simulink model "TVModel_Simulation_21"  (R2021b)
settings: Solver=FixedStepDiscrete  StartTime=0.0  StopTime=250  FixedStep=0.02  MaxStep=0.01  RelTol=1e-3
undefined symbols (not defined in the file or in its folder): MB, TV, TV_OLD
libraries: simulink x22, simulink_extras x14, eeGeneralControl x13, slpidlib x8, fuzblock x4, controlLib x4, cstblocks x3, dspstat3 x2, eeSlidingModeController x1, sharedTrackingLibrary x1
(part 7 of 9)

== matlab function TVModel_Simulation_21/Subsystem/Subsystem1/Torque Distribution/MPC/ PRE LUDO/Cross Check1 ==
  data: ubu input; param input; ubu output; lbu input; lbu output
function [ubu,lbu] = fcn(ubu,param,lbu)
flag = param(1);
ubu_target = param(2:5);
lbu_target = param(6:9);
lbu_max = param(10);
switch flag
    case 0 %% Check cross between bounds
        for i = 1 : 4
            if lbu(i) > ubu(i)
               lbu(i) = ubu(i) - lbu_max;
            end
        end
    case 1 %% Check for low YRD Accelerating
        for i = 1 :4
            ubu(i) = ubu_target(i);
            lbu(i) = 0;
        end
    case 2 %% Check for low YRD Braking
        for i = 1:4
            lbu(i) = lbu_target(i);
            ubu(i) = 0;
        end
    case 3 %% Overlapping
        for i = 1:4
            lbu(i) = 0;
            ubu(i) = 0;
        end
end

== matlab function TVModel_Simulation_21/Subsystem/Subsystem1/Torque Distribution/MPC/USEFUL STUFFFF/Extended Kalman Filter/state_update_kalman_simulink/f(x,u) ==
  data: x input; u input; xout output
function xout = state_update_kalman_simulink(x,u)

%% ~~~~~~~~~~~~~~~~~~~~~~~~~~~~~ Intro ~~~~~~~~~~~~~~~~~~~~~~~~~~~~~~~~~~~~
dt = 1/50;
%% ~~~~~~~~~~~~~~~~~~~~~~~~ Car parameters ~~~~~~~~~~~~~~~~~~~~~~~~~~~~~~~~
xout = zeros(3,1);
% ~~~~~~~~~~~~~~~~~~~~~~~~ General Parameters ~~~~~~~~~~~~~~~~~~~~~~~~~~~~~
g   = 9.81;            % [m/s^2]                          
wd  = 0.5;             % [~]         
wb  = 1.53;            % [~]          
tf  = 1.27;            % [m]          
tr  = 1.27;            % [m]          
m   = 195+75;          % [Kg]            
Iz  = 120;             % [Kg*m^2]         
a   = wb*wd;           % [m]            
b   = wb - a;          % [m]            
hcog = 0.29;           % [m]           
Fzf  = m*g/2*(wd);     % [N]                 
Fzr  = m*g/2*(1-wd);   % [N]                   
tau = 13.5;            % [~]          
rs  = 0.235;           % [m]           

% ~~~~~~~~~~~~~~~~~~~~~~~~~~~ Aero parameters ~~~~~~~~~~~~~~~~~~~~~~~~~~~~~
wbaero = 0.5542;       % [~]           
hcop = 0.576;          % [m]      
rho = 1.225;           % [Kg/m^3]     
CdA = 1.708;           % [m]     
ClA = 5.14;            % [m]    

% ~~~~~~~~~~~~~~~~~~~~~~~~~~ Other parameters ~~~~~~~~~~~~~~~~~~~~~~~~~~~~~

% ~~~~~~~~~~~~~~~~~~~~~~~~~~~ Set up states  ~~~~~~~~~~~~~~~~~~~~~~~~~~~~~~
vx = x(1);
vy = x(2);
r  = x(3);

% ~~~~~~~~~~~~~~~~~~~~~~~~~~~ Set up parameters ~~~~~~~~~~~~~~~~~~~~~~~~~~~
% delta    = u(1);
% kappa_FL = u(2);
% kappa_FR = u(3);
% kappa_RL = u(4);
% kappa_RR = u(5);
% Tbrk_FL  = u(6);
% Tbrk_FR  = u(7);
% Tbrk_RL  = u(8);
% Tbrk_RR  = u(9);
% ay       = u(10);
% ax       = u(11);
% T_FL     = u(12);
% T_FR     = u(13);
% T_RL     = u(14);
% T_RR     = u(15);

delta    = u(1);
kappa_FL = u(2);
kappa_FR = u(3);
kappa_RL = u(4);
kappa_RR = u(5);
T_FL     = u(6);
T_FR     = u(7);
T_RL     = u(8);
T_RR     = u(9);

ax = 0; ay = 0;
Tbrk_FL  = 0;
Tbrk_FR  = 0;
Tbrk_RL  = 0;
Tbrk_RR  = 0;
%% ~~~~~~~~~~~~~~~~~~~~~~~~~~ System Dynamics ~~~~~~~~~~~~~~~~~~~~~~~~~~~~~~

% ~~~~~~~~~~~~~~~~~~~~~~~~~~~ Aerodynamics ~~~~~~~~~~~~~~~~~~~~~~~~~~~~~~~~
Faerox = 0.5*rho*CdA*vx^2;
Faeroz = 0.5*rho*ClA*vx^2;

% ~~~~~~~~~~~~~~~~~~~~~~~~~~~ Slip Angles ~~~~~~~~~~~~~~~~~~~~~~~~~~~~~~~~~
alpha_FL =  (((vy + r*a)./(vx - r*tf/2)) - delta);
alpha_FR =  (((vy + r*a)./(vx + r*tf/2)) - delta);
alpha_RL =  (((vy - r*b)./(vx - r*tr/2)));     
alpha_RR =  (((vy - r*b)./(vx + r*tr/2)));     

% ~~~~~~~~~~~~~~~~~~~~~~~~~~~ Vertical loads ~~~~~~~~~~~~~~~~~~~~~~~~~~~~~~
Fz_FL = Fzf - 0.5*(m/tf*hcog).*ay + 0.5*Faeroz*wbaero - 0.5*Faerox/wb*hcop - 0.5*(m/wb*hcog).*ax;
Fz_FR = Fzf + 0.5*(m/tf*hcog).*ay + 0.5*Faeroz*wbaero - 0.5*Faerox/wb*hcop - 0.5*(m/wb*hcog).*ax;
Fz_RL = Fzr - 0.5*(m/tr*hcog).*ay + 0.5*Faeroz*(1-wbaero) + 0.5*Faerox/wb*hcop + 0.5*(m/wb*hcog).*ax;
Fz_RR = Fzr + 0.5*(m/tr*hcog).*ay + 0.5*Faeroz*(1-wbaero) + 0.5*Faerox/wb*hcop + 0.5*(m/wb*hcog).*ax;

% ~~~~~~~~~~~~~~~~~~~~~~~~~~ Lateral forces ~~~~~~~~~~~~~~~~~~~~~~~~~~~~~~~
muY = 1.5;
Fy_FL = (cos(0.95064*atan((41.4696*(kappa_FL - 0.00000078224999999999995925481499625675*Fz_FL + 0.00056678999999999995877686398415563))/((13.456699999999999661781657778192*alpha_FL - 0.51027806399999998717476046294905)^2 + 1.0)^(1/2) + (0.0012906*Fz_FL - 2.3215)*(atan((41.4696*(kappa_FL - 0.00000078224999999999995925481499625675*Fz_FL + 0.00056678999999999995877686398415563))/((13.456699999999999661781657778192*alpha_FL - 0.51027806399999998717476046294905)^2 + 1.0)^(1/2)) - (41.4696*(kappa_FL - 0.00000078224999999999995925481499625675*Fz_FL + 0.00056678999999999995877686398415563))/((13.456699999999999661781657778192*alpha_FL - 0.51027806399999998717476046294905)^2 + 1.0)^(1/2))))*(0.93*Fz_FL*(0.000071017999999999997795541162304289*Fz_FL - 0.14887799999999999779554116230429) - 0.93*Fz_FL*(0.00074656*Fz_FL + 0.37814) + Fz_FL*muY*sin(1.1962*atan((28888.097815192522084544179961085*sin(2.0*atan(0.00077863498204218704389788477193347*Fz_FL))*(0.000001140900000000000030428437547414*Fz_FL - 1.0*alpha_FL + (0.93*Fz_FL*(0.00074656*Fz_FL + 0.37814) + 1.1538900000000000822808488010196*Fz_FL*(0.00023917*Fz_FL - 1.57477))/(28888.097815192522084544179961085*sin(2.0*atan(0.00077863498204218704389788477193347*Fz_FL)) - 0.01) + 0.0023905000000000000467265115489113))/(1.1962*Fz_FL*muY + 0.01) - 1.0*(atan((28888.097815192522084544179961085*sin(2.0*atan(0.00077863498204218704389788477193347*Fz_FL))*(0.000001140900000000000030428437547414*Fz_FL - 1.0*alpha_FL + (0.93*Fz_FL*(0.00074656*Fz_FL + 0.37814) + 1.1538900000000000822808488010196*Fz_FL*(0.00023917*Fz_FL - 1.57477))/(28888.097815192522084544179961085*sin(2.0*atan(0.00077863498204218704389788477193347*Fz_FL)) - 0.01) + 0.0023905000000000000467265115489113))/(1.1962*Fz_FL*muY + 0.01)) - (28888.097815192522084544179961085*sin(2.0*atan(0.00077863498204218704389788477193347*Fz_FL))*(0.000001140900000000000030428437547414*Fz_FL - 1.0*alpha_FL + (0.93*Fz_FL*(0.00074656*Fz_FL + 0.37814) + 1.1538900000000000822808488010196*Fz_FL*(0.00023917*Fz_FL - 1.57477))/(28888.097815192522084544179961085*sin(2.0*atan(0.00077863498204218704389788477193347*Fz_FL)) - 0.01) + 0.0023905000000000000467265115489113))/(1.1962*Fz_FL*muY + 0.01))*(0.000039933999999999997276844965199416*Fz_FL - 0.52068399999999999727684496519942)*(0.47036*sign(0.000001140900000000000030428437547414*Fz_FL - 1.0*alpha_FL + (0.93*Fz_FL*(0.00074656*Fz_FL + 0.37814) + 1.1538900000000000822808488010196*Fz_FL*(0.00023917*Fz_FL - 1.57477))/(28888.097815192522084544179961085*sin(2.0*atan(0.00077863498204218704389788477193347*Fz_FL)) - 0.01) + 0.0023905000000000000467265115489113) - 7.9286)))))/cos(0.95064*atan((41.4696*(0.00000078224999999999995925481499625675*Fz_FL - 0.00056678999999999995877686398415563))/((13.456699999999999661781657778192*alpha_FL - 0.51027806399999998717476046294905)^2 + 1.0)^(1/2) + (0.0012906*Fz_FL - 2.3215)*(atan((41.4696*(0.00000078224999999999995925481499625675*Fz_FL - 0.00056678999999999995877686398415563))/((13.456699999999999661781657778192*alpha_FL - 0.51027806399999998717476046294905)^2 + 1.0)^(1/2)) - (41.4696*(0.00000078224999999999995925481499625675*Fz_FL - 0.00056678999999999995877686398415563))/((13.456699999999999661781657778192*alpha_FL - 0.51027806399999998717476046294905)^2 + 1.0)^(1/2)))) - (1.0*Fz_FL*muY*sin(1.9085*atan(16.5046*kappa_FL))*(0.0000027179999999999999299449271461526*Fz_FL - 1.1553830000000000000737188088351))/(225.17103248999997449603881705116*alpha_FL^2 + 1.0)^(1/2) + 400;
Fy_FR = (cos(0.95064*atan((41.4696*(kappa_FR - 0.00000078224999999999995925481499625675*Fz_FR + 0.00056678999999999995877686398415563))/((13.456699999999999661781657778192*alpha_FR - 0.51027806399999998717476046294905)^2 + 1.0)^(1/2) + (0.0012906*Fz_FR - 2.3215)*(atan((41.4696*(kappa_FR - 0.00000078224999999999995925481499625675*Fz_FR + 0.00056678999999999995877686398415563))/((13.456699999999999661781657778192*alpha_FR - 0.51027806399999998717476046294905)^2 + 1.0)^(1/2)) - (41.4696*(kappa_FR - 0.00000078224999999999995925481499625675*Fz_FR + 0.00056678999999999995877686398415563))/((13.456699999999999661781657778192*alpha_FR - 0.51027806399999998717476046294905)^2 + 1.0)^(1/2))))*(0.93*Fz_FR*(0.000071017999999999997795541162304289*Fz_FR - 0.14887799999999999779554116230429) - 0.93*Fz_FR*(0.00074656*Fz_FR + 0.37814) + Fz_FR*muY*sin(1.1962*atan((28888.097815192522084544179961085*sin(2.0*atan(0.00077863498204218704389788477193347*Fz_FR))*(0.000001140900000000000030428437547414*Fz_FR - 1.0*alpha_FR + (0.93*Fz_FR*(0.00074656*Fz_FR + 0.37814) + 1.1538900000000000822808488010196*Fz_FR*(0.00023917*Fz_FR - 1.57477))/(28888.097815192522084544179961085*sin(2.0*atan(0.00077863498204218704389788477193347*Fz_FR)) - 0.01) + 0.0023905000000000000467265115489113))/(1.1962*Fz_FR*muY + 0.01) - 1.0*(atan((28888.097815192522084544179961085*sin(2.0*atan(0.00077863498204218704389788477193347*Fz_FR))*(0.000001140900000000000030428437547414*Fz_FR - 1.0*alpha_FR + (0.93*Fz_FR*(0.00074656*Fz_FR + 0.37814) + 1.1538900000000000822808488010196*Fz_FR*(0.00023917*Fz_FR - 1.57477))/(28888.097815192522084544179961085*sin(2.0*atan(0.00077863498204218704389788477193347*Fz_FR)) - 0.01) + 0.0023905000000000000467265115489113))/(1.1962*Fz_FR*muY + 0.01)) - (28888.097815192522084544179961085*sin(2.0*atan(0.00077863498204218704389788477193347*Fz_FR))*(0.000001140900000000000030428437547414*Fz_FR - 1.0*alpha_FR + (0.93*Fz_FR*(0.00074656*Fz_FR + 0.37814) + 1.1538900000000000822808488010196*Fz_FR*(0.00023917*Fz_FR - 1.57477))/(28888.097815192522084544179961085*sin(2.0*atan(0.00077863498204218704389788477193347*Fz_FR)) - 0.01) + 0.0023905000000000000467265115489113))/(1.1962*Fz_FR*muY + 0.01))*(0.000039933999999999997276844965199416*Fz_FR - 0.52068399999999999727684496519942)*(0.47036*sign(0.000001140900000000000030428437547414*Fz_FR - 1.0*alpha_FR + (0.93*Fz_FR*(0.00074656*Fz_FR + 0.37814) + 1.1538900000000000822808488010196*Fz_FR*(0.00023917*Fz_FR - 1.57477))/(28888.097815192522084544179961085*sin(2.0*atan(0.00077863498204218704389788477193347*Fz_FR)) - 0.01) + 0.0023905000000000000467265115489113) - 7.9286)))))/cos(0.95064*atan((41.4696*(0.00000078224999999999995925481499625675*Fz_FR - 0.00056678999999999995877686398415563))/((13.456699999999999661781657778192*alpha_FR - 0.51027806399999998717476046294905)^2 + 1.0)^(1/2) + (0.0012906*Fz_FR - 2.3215)*(atan((41.4696*(0.00000078224999999999995925481499625675*Fz_FR - 0.00056678999999999995877686398415563))/((13.456699999999999661781657778192*alpha_FR - 0.51027806399999998717476046294905)^2 + 1.0)^(1/2)) - (41.4696*(0.00000078224999999999995925481499625675*Fz_FR - 0.00056678999999999995877686398415563))/((13.456699999999999661781657778192*alpha_FR - 0.51027806399999998717476046294905)^2 + 1.0)^(1/2)))) - (1.0*Fz_FR*muY*sin(1.9085*atan(16.5046*kappa_FR))*(0.0000027179999999999999299449271461526*Fz_FR - 1.1553830000000000000737188088351))/(225.17103248999997449603881705116*alpha_FR^2 + 1.0)^(1/2) + 400;
Fy_RL = (cos(0.95064*atan((41.4696*(kappa_RL - 0.00000078224999999999995925481499625675*Fz_RL + 0.00056678999999999995877686398415563))/((13.456699999999999661781657778192*alpha_RL - 0.51027806399999998717476046294905)^2 + 1.0)^(1/2) + (0.0012906*Fz_RL - 2.3215)*(atan((41.4696*(kappa_RL - 0.00000078224999999999995925481499625675*Fz_RL + 0.00056678999999999995877686398415563))/((13.456699999999999661781657778192*alpha_RL - 0.51027806399999998717476046294905)^2 + 1.0)^(1/2)) - (41.4696*(kappa_RL - 0.00000078224999999999995925481499625675*Fz_RL + 0.00056678999999999995877686398415563))/((13.456699999999999661781657778192*alpha_RL - 0.51027806399999998717476046294905)^2 + 1.0)^(1/2))))*(0.93*Fz_RL*(0.000071017999999999997795541162304289*Fz_RL - 0.14887799999999999779554116230429) - 0.93*Fz_RL*(0.00074656*Fz_RL + 0.37814) + Fz_RL*muY*sin(1.1962*atan((28888.097815192522084544179961085*sin(2.0*atan(0.00077863498204218704389788477193347*Fz_RL))*(0.000001140900000000000030428437547414*Fz_RL - 1.0*alpha_RL + (0.93*Fz_RL*(0.00074656*Fz_RL + 0.37814) + 1.1538900000000000822808488010196*Fz_RL*(0.00023917*Fz_RL - 1.57477))/(28888.097815192522084544179961085*sin(2.0*atan(0.00077863498204218704389788477193347*Fz_RL)) - 0.01) + 0.0023905000000000000467265115489113))/(1.1962*Fz_RL*muY + 0.01) - 1.0*(atan((28888.097815192522084544179961085*sin(2.0*atan(0.00077863498204218704389788477193347*Fz_RL))*(0.000001140900000000000030428437547414*Fz_RL - 1.0*alpha_RL + (0.93*Fz_RL*(0.00074656*Fz_RL + 0.37814) + 1.1538900000000000822808488010196*Fz_RL*(0.00023917*Fz_RL - 1.57477))/(28888.097815192522084544179961085*sin(2.0*atan(0.00077863498204218704389788477193347*Fz_RL)) - 0.01) + 0.0023905000000000000467265115489113))/(1.1962*Fz_RL*muY + 0.01)) - (28888.097815192522084544179961085*sin(2.0*atan(0.00077863498204218704389788477193347*Fz_RL))*(0.000001140900000000000030428437547414*Fz_RL - 1.0*alpha_RL + (0.93*Fz_RL*(0.00074656*Fz_RL + 0.37814) + 1.1538900000000000822808488010196*Fz_RL*(0.00023917*Fz_RL - 1.57477))/(28888.097815192522084544179961085*sin(2.0*atan(0.00077863498204218704389788477193347*Fz_RL)) - 0.01) + 0.0023905000000000000467265115489113))/(1.1962*Fz_RL*muY + 0.01))*(0.000039933999999999997276844965199416*Fz_RL - 0.52068399999999999727684496519942)*(0.47036*sign(0.000001140900000000000030428437547414*Fz_RL - 1.0*alpha_RL + (0.93*Fz_RL*(0.00074656*Fz_RL + 0.37814) + 1.1538900000000000822808488010196*Fz_RL*(0.00023917*Fz_RL - 1.57477))/(28888.097815192522084544179961085*sin(2.0*atan(0.00077863498204218704389788477193347*Fz_RL)) - 0.01) + 0.0023905000000000000467265115489113) - 7.9286)))))/cos(0.95064*atan((41.4696*(0.00000078224999999999995925481499625675*Fz_RL - 0.00056678999999999995877686398415563))/((13.456699999999999661781657778192*alpha_RL - 0.51027806399999998717476046294905)^2 + 1.0)^(1/2) + (0.0012906*Fz_RL - 2.3215)*(atan((41.4696*(0.00000078224999999999995925481499625675*Fz_RL - 0.00056678999999999995877686398415563))/((13.456699999999999661781657778192*alpha_RL - 0.51027806399999998717476046294905)^2 + 1.0)^(1/2)) - (41.4696*(0.00000078224999999999995925481499625675*Fz_RL - 0.00056678999999999995877686398415563))/((13.456699999999999661781657778192*alpha_RL - 0.51027806399999998717476046294905)^2 + 1.0)^(1/2)))) - (1.0*Fz_RL*muY*sin(1.9085*atan(16.5046*kappa_RL))*(0.0000027179999999999999299449271461526*Fz_RL - 1.1553830000000000000737188088351))/(225.17103248999997449603881705116*alpha_RL^2 + 1.0)^(1/2) + 400;
Fy_RR = (cos(0.95064*atan((41.4696*(kappa_RR - 0.00000078224999999999995925481499625675*Fz_RR + 0.00056678999999999995877686398415563))/((13.456699999999999661781657778192*alpha_RR - 0.51027806399999998717476046294905)^2 + 1.0)^(1/2) + (0.0012906*Fz_RR - 2.3215)*(atan((41.4696*(kappa_RR - 0.00000078224999999999995925481499625675*Fz_RR + 0.00056678999999999995877686398415563))/((13.456699999999999661781657778192*alpha_RR - 0.51027806399999998717476046294905)^2 + 1.0)^(1/2)) - (41.4696*(kappa_RR - 0.00000078224999999999995925481499625675*Fz_RR + 0.00056678999999999995877686398415563))/((13.456699999999999661781657778192*alpha_RR - 0.51027806399999998717476046294905)^2 + 1.0)^(1/2))))*(0.93*Fz_RR*(0.000071017999999999997795541162304289*Fz_RR - 0.14887799999999999779554116230429) - 0.93*Fz_RR*(0.00074656*Fz_RR + 0.37814) + Fz_RR*muY*sin(1.1962*atan((28888.097815192522084544179961085*sin(2.0*atan(0.00077863498204218704389788477193347*Fz_RR))*(0.000001140900000000000030428437547414*Fz_RR - 1.0*alpha_RR + (0.93*Fz_RR*(0.00074656*Fz_RR + 0.37814) + 1.1538900000000000822808488010196*Fz_RR*(0.00023917*Fz_RR - 1.57477))/(28888.097815192522084544179961085*sin(2.0*atan(0.00077863498204218704389788477193347*Fz_RR)) - 0.01) + 0.0023905000000000000467265115489113))/(1.1962*Fz_RR*muY + 0.01) - 1.0*(atan((28888.097815192522084544179961085*sin(2.0*atan(0.00077863498204218704389788477193347*Fz_RR))*(0.000001140900000000000030428437547414*Fz_RR - 1.0*alpha_RR + (0.93*Fz_RR*(0.00074656*Fz_RR + 0.37814) + 1.1538900000000000822808488010196*Fz_RR*(0.00023917*Fz_RR - 1.57477))/(28888.097815192522084544179961085*sin(2.0*atan(0.00077863498204218704389788477193347*Fz_RR)) - 0.01) + 0.0023905000000000000467265115489113))/(1.1962*Fz_RR*muY + 0.01)) - (28888.097815192522084544179961085*sin(2.0*atan(0.00077863498204218704389788477193347*Fz_RR))*(0.000001140900000000000030428437547414*Fz_RR - 1.0*alpha_RR + (0.93*Fz_RR*(0.00074656*Fz_RR + 0.37814) + 1.1538900000000000822808488010196*Fz_RR*(0.00023917*Fz_RR - 1.57477))/(28888.097815192522084544179961085*sin(2.0*atan(0.00077863498204218704389788477193347*Fz_RR)) - 0.01) + 0.0023905000000000000467265115489113))/(1.1962*Fz_RR*muY + 0.01))*(0.000039933999999999997276844965199416*Fz_RR - 0.52068399999999999727684496519942)*(0.47036*sign(0.000001140900000000000030428437547414*Fz_RR - 1.0*alpha_RR + (0.93*Fz_RR*(0.00074656*Fz_RR + 0.37814) + 1.1538900000000000822808488010196*Fz_RR*(0.00023917*Fz_RR - 1.57477))/(28888.097815192522084544179961085*sin(2.0*atan(0.00077863498204218704389788477193347*Fz_RR)) - 0.01) + 0.0023905000000000000467265115489113) - 7.9286)))))/cos(0.95064*atan((41.4696*(0.00000078224999999999995925481499625675*Fz_RR - 0.00056678999999999995877686398415563))/((13.456699999999999661781657778192*alpha_RR - 0.51027806399999998717476046294905)^2 + 1.0)^(1/2) + (0.0012906*Fz_RR - 2.3215)*(atan((41.4696*(0.00000078224999999999995925481499625675*Fz_RR - 0.00056678999999999995877686398415563))/((13.456699999999999661781657778192*alpha_RR - 0.51027806399999998717476046294905)^2 + 1.0)^(1/2)) - (41.4696*(0.00000078224999999999995925481499625675*Fz_RR - 0.00056678999999999995877686398415563))/((13.456699999999999661781657778192*alpha_RR - 0.51027806399999998717476046294905)^2 + 1.0)^(1/2)))) - (1.0*Fz_RR*muY*sin(1.9085*atan(16.5046*kappa_RR))*(0.0000027179999999999999299449271461526*Fz_RR - 1.1553830000000000000737188088351))/(225.17103248999997449603881705116*alpha_RR^2 + 1.0)^(1/2) + 400;

% ~~~~~~~~~~~~~~~~~~~~~~~~~~ Longitudinal forces ~~~~~~~~~~~~~~~~~~~~~~~~~~
Fx_FL = (T_FL.*tau - Tbrk_FL)/rs;
Fx_FR = (T_FR.*tau - Tbrk_FR)/rs;
Fx_RL = (T_RL.*tau - Tbrk_RL)/rs;
Fx_RR = (T_RR.*tau - Tbrk_RR)/rs;

% ~~~~~~~~~~~~~~~~~~~~~~~~~~~ E.o.M. Balance ~~~~~~~~~~~~~~~~~~~~~~~~~~~~~~
X1 = (Fx_FL + Fx_FR).*cos(delta) - (Fy_FL + Fy_FR).*sin(delta);
X2 = Fx_RL + Fx_RR;
deltaX1 = ((Fx_FR - Fx_FL).*cos(delta) - (Fy_FR - Fy_FL).*sin(delta))/2;
deltaX2 = (Fx_RR - Fx_RL)/2;

Y1 = (Fy_FL + Fy_FR).*cos(delta) + (Fx_FL + Fx_FR).*sin(delta);
Y2 = Fy_RL + Fy_RR;

X = X1 + X2 - Faerox;
Y = Y1 + Y2;
N = Y1*a - Y2*b + deltaX1*tf + deltaX2*tr;

% ~~~~~~~~~~~~~~~~~~~~~~~~~~~ System Dynamics f(x,u) ~~~~~~~~~~~~~~~~~~~~~~
xout(1) =  1/m.*(X + vy.*r)*dt + x(1);
xout(2) =  1/m.*(Y - vx.*r)*dt + x(2);
xout(3) =  1/Iz.*(N)*dt + x(3);
end

== matlab function TVModel_Simulation_21/Subsystem/Subsystem1/Torque Distribution/MPC/USEFUL STUFFFF/Extended Kalman Filter/measurement_kalman_simulink/h(x) ==
  data: x input; y output
function y = measurement_kalman_simulink(x)

y = zeros(3,1);
y(1) = x(1);
y(2) = x(2);
y(3) = x(3);

end

== stateflow chart TVModel_Simulation_21/Subsystem/Subsystem1/Slip Control/Traction Control/TC_Activation_Logic ==
  state TS_ON
    state TC_OFF
      en,du:
      t_max_pid(1:4) = t_limit_positive(1:4);
    state TC_ON
      state FL [parallel]
        settings: executionOrder=1
        state TC_INACTIVE
          en:
          t_max_pid(1) = t_limit_positive(1);
          du:
          t_max_pid(1) = t_limit_positive(1);
        state TC_ACTIVE
          en:
          t_max_pid(1) = abs(t_actual(1));
          du:
          t_max_pid(1) = t_max_pid(1)+t_pid(1);
        (default) -> TS_ON.TC_ON.FL.TC_INACTIVE
        TS_ON.TC_ON.FL.TC_INACTIVE -> TS_ON.TC_ON.FL.TC_ACTIVE : [slip_ratio(1) >= slip_ratio_target]
        TS_ON.TC_ON.FL.TC_ACTIVE -> TS_ON.TC_ON.FL.TC_INACTIVE : [slip_ratio(1) < slip_ratio_target*0.3]
      state FR [parallel]
        settings: executionOrder=2
        state TC_ACTIVE
          en:
          t_max_pid(2) = abs(t_actual(2));
          du:
          t_max_pid(2) = t_max_pid(2)+t_pid(2);
        state TC_INACTIVE
          en:
          t_max_pid(2) = t_limit_positive(2);
          du:
          t_max_pid(2) = t_limit_positive(2);
        (default) -> TS_ON.TC_ON.FR.TC_INACTIVE
        TS_ON.TC_ON.FR.TC_INACTIVE -> TS_ON.TC_ON.FR.TC_ACTIVE : [slip_ratio(2) >= slip_ratio_target]
        TS_ON.TC_ON.FR.TC_ACTIVE -> TS_ON.TC_ON.FR.TC_INACTIVE : [slip_ratio(2) < slip_ratio_target*0.3]
      state RL [parallel]
        settings: executionOrder=3
        state TC_INACTIVE
          en:
          t_max_pid(3) = t_limit_positive(3);
          du:
          t_max_pid(3) = t_limit_positive(3);
        state TC_ACTIVE
          en:
          t_max_pid(3) = abs(t_actual(3));
          du:
          t_max_pid(3) = t_max_pid(3)+t_pid(3);
        (default) -> TS_ON.TC_ON.RL.TC_INACTIVE
        TS_ON.TC_ON.RL.TC_INACTIVE -> TS_ON.TC_ON.RL.TC_ACTIVE : [slip_ratio(3) >= slip_ratio_target]
        TS_ON.TC_ON.RL.TC_ACTIVE -> TS_ON.TC_ON.RL.TC_INACTIVE : [slip_ratio(3) < slip_ratio_target*0.3]
      state RR [parallel]
        settings: executionOrder=4
        state TC_ACTIVE
          en:
          t_max_pid(4) = abs(t_actual(4));
          du:
          t_max_pid(4) = t_max_pid(4)+t_pid(4);
        state TC_INACTIVE
          en:
          t_max_pid(4) = t_limit_positive(4);
          du:
          t_max_pid(4) = t_limit_positive(4);
        (default) -> TS_ON.TC_ON.RR.TC_INACTIVE
        TS_ON.TC_ON.RR.TC_INACTIVE -> TS_ON.TC_ON.RR.TC_ACTIVE : [slip_ratio(4) >= slip_ratio_target]
        TS_ON.TC_ON.RR.TC_ACTIVE -> TS_ON.TC_ON.RR.TC_INACTIVE : [slip_ratio(4) < slip_ratio_target*0.3]
    (default) -> TC_OFF
    TC_ON -> TC_OFF : [tc_flag == 0]
    TC_OFF -> TC_ON : [tc_flag == 1]
  state TS_OFF
    en:
    t_max_pid(1:4) = zeros(4,1);
  (default) -> TS_OFF
  TS_OFF -> TS_ON : [rtd_flag == 1]
  TS_ON -> TS_OFF : [rtd_flag == 0]
  data: t_pid input; t_actual input; rtd_flag input; tc_flag input; t_max_pid output =zeros(4, 1); t_limit_positive input; slip_ratio input; slip_ratio_target input

== matlab function TVModel_Simulation_21/Subsystem/Subsystem1/Slip Control/Traction Control/TC/MATLAB Function1 ==
  data: vx input; T output; kappa input; Fz input; IN input; omega_p input; alpha input
function T = fcn(vx,kappa,Fz,IN,omega_p,alpha)

LMU = 0.8;
J_wheel = 2e5/1e6;
rs = 0.235;
m = 270/4;
tau = 13.5;
dt = 0.02;
g = 9.81;

% @(Fz,LMUX,kappa)
% Old tire
% muX = ((Fz.^2.*LMUX)./1.0e+4-Fz.*LMUX.*sin(atan((Fz.*5.946e-5-6.5736e-1).*(sign(Fz.*(-1.5696e-6)+kappa+6.665e-4).*5.242e-1+1.0).*(atan((Fz.*exp(Fz.*(-1.3455e-5)+1.3455e-2).*(Fz.*(3.0./2.0e+2)+6.77e+2./1.0e+1).*(Fz.*(-1.5696e-6)+kappa+6.665e-4).*(3.33e+2./4.0e+2))./(Fz.*LMUX.*2.5847808+1.0./1.0e+2))-(Fz.*exp(Fz.*(-1.3455e-5)+1.3455e-2).*(Fz.*(3.0./2.0e+2)+6.77e+2./1.0e+1).*(Fz.*(-1.5696e-6)+kappa+6.665e-4).*(3.33e+2./4.0e+2))./(Fz.*LMUX.*2.5847808+1.0./1.0e+2))-(Fz.*exp(Fz.*(-1.3455e-5)+1.3455e-2).*(Fz.*(3.0./2.0e+2)+6.77e+2./1.0e+1).*(Fz.*(-1.5696e-6)+kappa+6.665e-4).*(3.33e+2./4.0e+2))./(Fz.*LMUX.*2.5847808+1.0./1.0e+2)).*(1.68e+2./1.25e+2)).*1.9232)./Fz;

% New tire
% muX = (1.0e-4.*Fz.^2.*LMU - 1.92.*Fz.*LMU.*sin(1.41.*atan(0.7.*(5.95e-5.*Fz - 0.657).*(0.524*sign(kappa - 1.57e-6.*Fz + 6.66e-4) + 1.0).*(atan((0.7.*Fz.*exp(0.0135 - 1.35e-5.*Fz).*(0.015.*Fz + 67.7).*(kappa - 1.57e-6.*Fz + 6.66e-4))./(2.71.*Fz.*LMU + 0.01)) - (0.7.*Fz.*exp(0.0135 - 1.35e-5.*Fz).*(0.015.*Fz + 67.7).*(kappa - 1.57e-6.*Fz + 6.66e-4))./(2.71.*Fz.*LMU + 0.01)) - (0.7.*Fz.*exp(0.0135 - 1.35e-5.*Fz).*(0.015.*Fz + 67.7).*(kappa - 1.57e-6.*Fz + 6.66e-4))./(2.71.*Fz.*LMU + 0.01))))./Fz;
% alpha = zeros(4,1);

muX_com = abs((cos(0.989.*atan((23.4.*(alpha - 0.00681))./(635.0.*kappa.^2 + 1.0).^(1/2) - 1.0.*(atan((23.4.*(alpha - 0.00681))./(635.0.*kappa.^2 + 1.0).^(1/2)) - (23.4.*(alpha - 0.00681))./(635.0.*kappa.^2 + 1.0).^(1/2)).*(2.08e-4.*Fz + 0.117))).*(1.0e-4.*Fz.^2.*LMU - 1.92.*Fz.*LMU.*sin(1.41.*atan(0.7.*(5.95e-5.*Fz - 0.657).*(0.524.*sign(kappa - 1.57e-6.*Fz + 6.66e-4) + 1.0).*(atan((0.7.*Fz.*exp(0.0135 - 1.35e-5.*Fz).*(0.015.*Fz + 67.7).*(kappa - 1.57e-6.*Fz + 6.66e-4))./(2.71.*Fz.*LMU + 0.01)) - (0.7.*Fz.*exp(0.0135 - 1.35e-5.*Fz).*(0.015.*Fz + 67.7).*(kappa - 1.57e-6.*Fz + 6.66e-4))./(2.71.*Fz.*LMU + 0.01)) - (0.7.*Fz.*exp(0.0135 - 1.35e-5.*Fz).*(0.015.*Fz + 67.7).*(kappa - 1.57e-6.*Fz + 6.66e-4))./(2.71.*Fz.*LMU + 0.01)))))./(Fz.*cos(0.989.*atan((atan(0.159./(635.0.*kappa.^2 + 1.0).^(1/2)) - 0.159./(635.0.*kappa.^2 + 1.0).^(1/2)).*(2.08e-4.*Fz + 0.117) - 0.159./(635.0.*kappa.^2 + 1.0).^(1/2)))));

% T_fb = kappa_p/vx;
% kappa_lim = 0.1*ones(4,1);
% 
% for i = 1 : 4
%     if kappa(i) < kappa_lim(i)
%        T_fb(i) = 0;
%     end
% end

T= (IN + ( (1-kappa)/m + rs^2/J_wheel ).*Fz.*muX_com).*J_wheel/rs/tau;

% eta = - omega_p*rs/g;

% T_ff_deceleration = (+rs.^2./J_wheel./g.*muX.*Fz - eta).*J_wheel.*g/rs/tau/2;

% alpha = 0.96;
% alpha = 1;

% T_ff = T_ff_slip*alpha + T_ff_deceleration*(1 - alpha);

end

== matlab function TVModel_Simulation_21/Subsystem/Subsystem1/Torque Distribution/MPC/USEFUL STUFFFF/Non-Linear Activation ==
  data: in_1 input; epsilon input; out output; in_2 input
function out = fcn(in_1,epsilon,in_2)

beta = 4;
epsilon = 1/(1 + (epsilon/(1-epsilon))^(-beta) );

out = in_1*epsilon + in_2*(1 - epsilon) ;

== stateflow chart TVModel_Simulation_21/Subsystem/Subsystem1/Torque Distribution/MPC/USEFUL STUFFFF/Chart ==
  state PID_on
    en:
    PID_flag = 1;
  state PID_off
    en:
    PID_flag = 0;
  (default) -> PID_on
  PID_on -> PID_off : [(front_wheels_steering-steer_threshold+semi_amplitude)/(2*semi_amplitude) < 1]
  PID_off -> PID_on : [(front_wheels_steering-steer_threshold+semi_amplitude)/(2*semi_amplitude) > 1]
  data: front_wheels_steering input; semi_amplitude input; PID_flag output; steer_threshold input

== matlab function TVModel_Simulation_21/Subsystem/Subsystem1/Torque Distribution/MPC/USEFUL STUFFFF/Yrd 0 When Steering 0/Linear Activation ==
  data: in_1 input; epsilon input; out output; in_2 input
function out = fcn(in_1,epsilon,in_2)

out = in_1*epsilon + in_2*(1 - epsilon) ;

== stateflow chart TVModel_Simulation_21/Subsystem/Subsystem1/Torque Distribution/MPC/Faults Detection/Overlap Chart ==
  state Stop
    en:
    torque_flag = 0;
  state Go
    en:
    torque_flag = 1;
  (default) -> Go
  Go -> Stop : [brake > 0]
  Stop -> Go : [(brake<=0.05 && throttle<0.05)]
  data: throttle input; brake input; torque_flag output

== matlab function TVModel_Simulation_21/Subsystem/Subsystem1/Torque Distribution/MPC/States Constraints/Cross Check ==
  data: ubx_in input; bounds input; ubx_out output size=4; lbx_in input; lbx_out output size=4; epsilon input; throttle input; brake input
function [ubx_out,lbx_out] = fcn(ubx_in,bounds,lbx_in,epsilon,throttle,brake)
    
    ubx_out = ubx_in;
    lbx_out = lbx_in;
    lbx_max = bounds(10);
    
    % cross between bounds
    switch epsilon
        case 1
            for i = 1 : 4
                if lbx_in(i) > ubx_in(i)
                   lbx_out(i) = ubx_in(i) - lbx_max;
                end
            end
        case 0
            if throttle > 0.05
               for i = 1 : 4
                   lbx_out(i) = 0;
               end
            elseif brake > 0.05
               for i = 1 : 4
                   ubx_out(i) = 0;
               end       
            else
            end
    end
end

== matlab function TVModel_Simulation_21/Subsystem/Subsystem1/Slip Control/Traction Control/TC/MATLAB Function2 ==
  data: T_max_controller input; T_max output; slip input; T_actual input; T_max_old input
function T_max = fcn(T_max_controller,slip,T_actual,T_max_old)

slip_target = 0.1*ones(4,1);
sDeact = 0.75;
T_max = zeros(4,1);

for i = 1:4 
    
    if slip(i) > slip_target(i)
        T_max(i) = T_max_controller(i);
    elseif T_actual(i) < T_max_old(i)*sDeact + 0.1;
        T_max(i) = T_max_old(i)+1;
        if T_max(i) > 21
           T_max(i) = 21;
        end
    else
        T_max(i) = T_max_controller(i);
    end
    
end

== matlab function TVModel_Simulation_21/Subsystem/Subsystem1/Torque Distribution/MPC/Weights Generation/MATLAB Function ==
  data: u input; y output; deltaAxle input
function y = fcn(u,deltaAxle)

Q = diag([u(1),u(2),u(3),u(4),u(5),u(6),u(7)]);
R = diag([u(8),u(9),u(10),u(11)]);
unscale = 50;
W = blkdiag(Q, R);
% 
% W(4,6) = -deltaAxle;
% W(6,4) = W(4,6);
% 
% W(5,7) = -deltaAxle;
% W(7,5) = W(5,7);

W = unscale*W;

y = W(:);

== matlab function TVModel_Simulation_21/Subsystem/Subsystem1/Torque Distribution/Reference Tracking/MATLAB Function ==
  data: LUT_brk input; brk input; YRD output; LUT_thr input
function YRD = fcn(LUT_brk,brk,LUT_thr)

YRD = LUT_brk*brk + LUT_thr*(1 - brk) ;

== matlab function TVModel_Simulation_21/Subsystem/Subsystem1/Torque Distribution/MPC/USEFUL STUFFFF/Subsystem/MATLAB Function ==
  data: T input; Tnew output; Plim input; Eta input; Omega input; Torque input; Omega_motors input; k output; fx output; brake_flag input
function [Tnew,k,fx] = fcn(T,Plim,Eta,Omega,Torque,Omega_motors,brake_flag)

Tnew = zeros(4,1);
fx = 10^3;
k      = 0;

exit   = 0;
dT     = 0;
eps    = 0.01;
h      = 0.3;
dT_new = 0;

eta_Plim = 1;

while exit == 0

    if brake_flag == 0;
        Tnew(1) = T(1) - dT;
        Tnew(2) = T(2) - dT;
        Tnew(3) = T(3) - dT;
        Tnew(4) = T(4) - dT;  
    
        eta = efficiency(Eta,Omega,Torque,Tnew,Omega_motors);
   

        for i = 1 : 4
            if Tnew(i) <= 0 
               Tnew(i) = 0;
            end
        end
    else
        Tnew(1) = T(1) + dT;
        Tnew(2) = T(2) + dT;
        Tnew(3) = T(3) + dT;
        Tnew(4) = T(4) + dT;  
    
        eta = efficiency(Eta,Omega,Torque,Tnew,Omega_motors);
   

        for i = 1 : 4
            if Tnew(i) >= 0 
               Tnew(i) = 0;
            end
        end
    end
%     eta1_hplus = efficiency(Eta,Omega,Torque,T1 - (dT + h),w1);
%     eta1_hminus = efficiency(Eta,Omega,Torque,T1 - (dT -h),w1);
%     eta2_hplus = efficiency(Eta,Omega,Torque,T2 - (dT + h),w2);
%     eta2_hminus = efficiency(Eta,Omega,Torque,T2 - (dT -h),w2);  
    fx = ( dot(Tnew./eta,Omega_motors') - Plim*eta_Plim );
    dT_new = dT + h;
    
%     fdotx = (-1/eta1/ ((eta1_hplus - eta1_hminus)/(2*h)) -1/eta2/ ((eta2_hplus - eta2_hminus)/(2*h)) );
%     dT_new = dT -  fx/fdotx;
    if k >= 100 || fx<0 || isnan(fx)
       exit = 1;
    else 
       dT = dT_new;
       k = k + 1;
    end

end

end

function eta = efficiency(Eta,Omega,Torque,T,w)    
         eta = interp2(Torque,Omega,Eta,abs(T),abs(w),"linear");
end

== matlab function TVModel_Simulation_21/Subsystem/Subsystem1/Slip Control/Traction Control/Slip Control/TC/MATLAB Function2 ==
  data: T_max_controller input; T_max output; slip input; slip_target input; T_actual input; T_max_old input
function T_max = fcn(T_max_controller,slip,slip_target,T_actual,T_max_old)

sDeact = 0.75;
T_max = zeros(4,1);

for i = 1:4 
    
    if slip(i) > slip_target(i)
        T_max(i) = T_max_controller(i);
    elseif T_actual(i) < T_max_old(i)*sDeact + 0.1;
        T_max(i) = T_max_old(i)+1;
        if T_max(i) > 21
           T_max(i) = 21;
        end
    else
        T_max(i) = T_max_controller(i);
    end
    
end

== matlab function TVModel_Simulation_21/Subsystem/Subsystem1/Torque Distribution/MPC/Faults Detection/Simple torque/No_TV/MATLAB Function ==
  data: T input; Tnew output; Plim input; Eta input; Omega input; Torque input; Omega_motors input; k output; fx output; brake_flag input
function [Tnew,k,fx] = fcn(T,Plim,Eta,Omega,Torque,Omega_motors,brake_flag)

Tnew = zeros(4,1);
fx = 10^3;
k      = 0;

exit   = 0;
dT     = 0;
eps    = 0.01;
h      = 0.3;
dT_new = 0;

eta_Plim = 1;

while exit == 0

    if brake_flag == 0;
        Tnew(1) = T(1) - dT;
        Tnew(2) = T(2) - dT;
        Tnew(3) = T(3) - dT;
        Tnew(4) = T(4) - dT;  
    
        eta = efficiency(Eta,Omega,Torque,Tnew,Omega_motors);
   

        for i = 1 : 4
            if Tnew(i) <= 0 
               Tnew(i) = 0;
            end
        end
    else
        Tnew(1) = T(1) + dT;
        Tnew(2) = T(2) + dT;
        Tnew(3) = T(3) + dT;
        Tnew(4) = T(4) + dT;  
    
        eta = efficiency(Eta,Omega,Torque,Tnew,Omega_motors);
   

        for i = 1 : 4
            if Tnew(i) >= 0 
               Tnew(i) = 0;
            end
        end
    end
%     eta1_hplus = efficiency(Eta,Omega,Torque,T1 - (dT + h),w1);
%     eta1_hminus = efficiency(Eta,Omega,Torque,T1 - (dT -h),w1);
%     eta2_hplus = efficiency(Eta,Omega,Torque,T2 - (dT + h),w2);
%     eta2_hminus = efficiency(Eta,Omega,Torque,T2 - (dT -h),w2);  
    fx = ( dot(Tnew./eta,Omega_motors') - Plim*eta_Plim );
    dT_new = dT + h;
    
%     fdotx = (-1/eta1/ ((eta1_hplus - eta1_hminus)/(2*h)) -1/eta2/ ((eta2_hplus - eta2_hminus)/(2*h)) );
%     dT_new = dT -  fx/fdotx;
    if k >= 100 || fx<0 || isnan(fx)
       exit = 1;
    else 
       dT = dT_new;
       k = k + 1;
    end

if isnan(k)
   k = 0;
end
if isnan(fx) 
   fx = 0;
end
if isnan(Tnew)
    Tnew = zeros(4,1);
end

end

end

function eta = efficiency(Eta,Omega,Torque,T,w)    
         eta = interp2(Torque,Omega,Eta,abs(T),abs(w),"linear");
end

== matlab function TVModel_Simulation_21/Subsystem/Subsystem1/Torque Distribution/MPC/Useful Calculations/MATLAB Function ==
  data: T input; y output; delta input
function y = fcn(T,delta)

tf = 1.27;
tr = 1.27;
a = 0.765;

delta_l = delta(1);
delta_r = delta(2);

y = sum(T.*[a.*sin(delta_l)-tf/2.*cos(delta_l);+a.*sin(delta_r)+tf/2*cos(delta_r);-tr/2;tr/2]);

== matlab function TVModel_Simulation_21/Subsystem/Subsystem1/Slip Control/Traction Control/ABS/MATLAB Function ==
  data: u_max_old input; vx input; u output; Fz input; kappa input
function u = linear_mpc(u_max_old,vx,Fz,kappa)

LMU = 0.8;
rs = 0.235;
Iw = 2e5/1e6;
dt = 0.2;
tau = 13.5;
dt = 0.02;
g = 9.81;

B = rs^2/Iw/vx*dt;

u = zeros(4,1);
u(1) = tc(u_max_old(1),vx,Fz(1),kappa(1));
u(2) = tc(u_max_old(2),vx,Fz(2),kappa(2));
u(3) = tc(u_max_old(3),vx,Fz(3),kappa(3));
u(4) = tc(u_max_old(4),vx,Fz(4),kappa(4));

end
% Astar = (0.0148*cos(0.989*atan((atan(0.159/(635.0*kappa^2 + 1.0)^(1/2)) - 0.159/(635.0*kappa^2 + 1.0)^(1/2))*(2.08e-4*Fz + 0.117) - 0.159/(635.0*kappa^2 + 1.0)^(1/2)))*(1.0e-4*Fz^2*LMU - 1.92*Fz*LMU*sin(1.41*atan((4.17e-5*Fz - 0.46)*(0.524*sign(kappa - 1.57e-6*Fz + 6.66e-4) + 1.0)*(atan((0.7*Fz*exp(0.0135 - 1.35e-5*Fz)*(0.015*Fz + 67.7)*(kappa - 1.57e-6*Fz + 6.66e-4))/(2.71*Fz*LMU + 0.01)) - (0.7*Fz*exp(0.0135 - 1.35e-5*Fz)*(0.015*Fz + 67.7)*(kappa - 1.57e-6*Fz + 6.66e-4))/(2.71*Fz*LMU + 0.01)) - (0.7*Fz*exp(0.0135 - 1.35e-5*Fz)*(0.015*Fz + 67.7)*(kappa - 1.57e-6*Fz + 6.66e-4))/(2.71*Fz*LMU + 0.01)))))/(vx*cos(0.989*atan(0.159/(635.0*kappa^2 + 1.0)^(1/2) - 1.0*(atan(0.159/(635.0*kappa^2 + 1.0)^(1/2)) - 0.159/(635.0*kappa^2 + 1.0)^(1/2))*(2.08e-4*Fz + 0.117)))) + (0.989*sin(0.989*atan((atan(0.159/(635.0*kappa^2 + 1.0)^(1/2)) - 0.159/(635.0*kappa^2 + 1.0)^(1/2))*(2.08e-4*Fz + 0.117) - 0.159/(635.0*kappa^2 + 1.0)^(1/2)))*(1.0e-4*Fz^2*LMU - 1.92*Fz*LMU*sin(1.41*atan((4.17e-5*Fz - 0.46)*(0.524*sign(kappa - 1.57e-6*Fz + 6.66e-4) + 1.0)*(atan((0.7*Fz*exp(0.0135 - 1.35e-5*Fz)*(0.015*Fz + 67.7)*(kappa - 1.57e-6*Fz + 6.66e-4))/(2.71*Fz*LMU + 0.01)) - (0.7*Fz*exp(0.0135 - 1.35e-5*Fz)*(0.015*Fz + 67.7)*(kappa - 1.57e-6*Fz + 6.66e-4))/(2.71*Fz*LMU + 0.01)) - (0.7*Fz*exp(0.0135 - 1.35e-5*Fz)*(0.015*Fz + 67.7)*(kappa - 1.57e-6*Fz + 6.66e-4))/(2.71*Fz*LMU + 0.01))))*((2.08e-4*Fz + 0.117)*((101.0*kappa)/(635.0*kappa^2 + 1.0)^(3/2) - (101.0*kappa)/((635.0*kappa^2 + 1.0)^(3/2)*(0.0254/(635.0*kappa^2 + 1.0) + 1.0))) + (101.0*kappa)/(635.0*kappa^2 + 1.0)^(3/2))*(rs^2/Iw - 0.0148*kappa + 0.0148))/(vx*cos(0.989*atan(0.159/(635.0*kappa^2 + 1.0)^(1/2) - 1.0*(atan(0.159/(635.0*kappa^2 + 1.0)^(1/2)) - 0.159/(635.0*kappa^2 + 1.0)^(1/2))*(2.08e-4*Fz + 0.117)))*(((atan(0.159/(635.0*kappa^2 + 1.0)^(1/2)) - 0.159/(635.0*kappa^2 + 1.0)^(1/2))*(2.08e-4*Fz + 0.117) - 0.159/(635.0*kappa^2 + 1.0)^(1/2))^2 + 1.0)) + (0.989*cos(0.989*atan((atan(0.159/(635.0*kappa^2 + 1.0)^(1/2)) - 0.159/(635.0*kappa^2 + 1.0)^(1/2))*(2.08e-4*Fz + 0.117) - 0.159/(635.0*kappa^2 + 1.0)^(1/2)))*sin(0.989*atan(0.159/(635.0*kappa^2 + 1.0)^(1/2) - 1.0*(atan(0.159/(635.0*kappa^2 + 1.0)^(1/2)) - 0.159/(635.0*kappa^2 + 1.0)^(1/2))*(2.08e-4*Fz + 0.117)))*(1.0e-4*Fz^2*LMU - 1.92*Fz*LMU*sin(1.41*atan((4.17e-5*Fz - 0.46)*(0.524*sign(kappa - 1.57e-6*Fz + 6.66e-4) + 1.0)*(atan((0.7*Fz*exp(0.0135 - 1.35e-5*Fz)*(0.015*Fz + 67.7)*(kappa - 1.57e-6*Fz + 6.66e-4))/(2.71*Fz*LMU + 0.01)) - (0.7*Fz*exp(0.0135 - 1.35e-5*Fz)*(0.015*Fz + 67.7)*(kappa - 1.57e-6*Fz + 6.66e-4))/(2.71*Fz*LMU + 0.01)) - (0.7*Fz*exp(0.0135 - 1.35e-5*Fz)*(0.015*Fz + 67.7)*(kappa - 1.57e-6*Fz + 6.66e-4))/(2.71*Fz*LMU + 0.01))))*((2.08e-4*Fz + 0.117)*((101.0*kappa)/(635.0*kappa^2 + 1.0)^(3/2) - (101.0*kappa)/((635.0*kappa^2 + 1.0)^(3/2)*(0.0253/(635.0*kappa^2 + 1.0) + 1.0))) + (101.0*kappa)/(635.0*kappa^2 + 1.0)^(3/2))*(rs^2/Iw - 0.0148*kappa + 0.0148))/(vx*cos(0.989*atan(0.159/(635.0*kappa^2 + 1.0)^(1/2) - 1.0*(atan(0.159/(635.0*kappa^2 + 1.0)^(1/2)) - 0.159/(635.0*kappa^2 + 1.0)^(1/2))*(2.08e-4*Fz + 0.117)))^2*((1.0*(atan(0.159/(635.0*kappa^2 + 1.0)^(1/2)) - 0.159/(635.0*kappa^2 + 1.0)^(1/2))*(2.08e-4*Fz + 0.117) - 0.159/(635.0*kappa^2 + 1.0)^(1/2))^2 + 1.0)) - (2.71*Fz*LMU*cos(1.41*atan((4.17e-5*Fz - 0.46)*(0.524*sign(kappa - 1.57e-6*Fz + 6.66e-4) + 1.0)*(atan((0.7*Fz*exp(0.0135 - 1.35e-5*Fz)*(0.015*Fz + 67.7)*(kappa - 1.57e-6*Fz + 6.66e-4))/(2.71*Fz*LMU + 0.01)) - (0.7*Fz*exp(0.0135 - 1.35e-5*Fz)*(0.015*Fz + 67.7)*(kappa - 1.57e-6*Fz + 6.66e-4))/(2.71*Fz*LMU + 0.01)) - (0.7*Fz*exp(0.0135 - 1.35e-5*Fz)*(0.015*Fz + 67.7)*(kappa - 1.57e-6*Fz + 6.66e-4))/(2.71*Fz*LMU + 0.01)))*cos(0.989*atan((atan(0.159/(635.0*kappa^2 + 1.0)^(1/2)) - 0.159/(635.0*kappa^2 + 1.0)^(1/2))*(2.08e-4*Fz + 0.117) - 0.159/(635.0*kappa^2 + 1.0)^(1/2)))*(((0.7*Fz*exp(0.0135 - 1.35e-5*Fz)*(0.015*Fz + 67.7))/(2.71*Fz*LMU + 0.01) - (0.7*Fz*exp(0.0135 - 1.35e-5*Fz)*(0.015*Fz + 67.7))/(((0.49*Fz^2*exp(0.027 - 2.7e-5*Fz)*(0.015*Fz + 67.7)^2*(kappa - 1.57e-6*Fz + 6.66e-4)^2)/(2.71*Fz*LMU + 0.01)^2 + 1.0)*(2.71*Fz*LMU + 0.01)))*(4.17e-5*Fz - 0.46)*(0.524*sign(kappa - 1.57e-6*Fz + 6.66e-4) + 1.0) - 1.05*dirac(kappa - 1.57e-6*Fz + 6.66e-4)*(4.17e-5*Fz - 0.46)*(atan((0.7*Fz*exp(0.0135 - 1.35e-5*Fz)*(0.015*Fz + 67.7)*(kappa - 1.57e-6*Fz + 6.66e-4))/(2.71*Fz*LMU + 0.01)) - (0.7*Fz*exp(0.0135 - 1.35e-5*Fz)*(0.015*Fz + 67.7)*(kappa - 1.57e-6*Fz + 6.66e-4))/(2.71*Fz*LMU + 0.01)) + (0.7*Fz*exp(0.0135 - 1.35e-5*Fz)*(0.015*Fz + 67.7))/(2.71*Fz*LMU + 0.01))*(rs^2/Iw - 0.0148*kappa + 0.0148))/(vx*cos(0.989*atan(0.159/(635.0*kappa^2 + 1.0)^(1/2) - 1.0*(atan(0.159/(635.0*kappa^2 + 1.0)^(1/2)) - 0.159/(635.0*kappa^2 + 1.0)^(1/2))*(2.08e-4*Fz + 0.117)))*(((4.17e-5*Fz - 0.46)*(0.524*sign(kappa - 1.57e-6*Fz + 6.66e-4) + 1.0)*(atan((0.7*Fz*exp(0.0135 - 1.35e-5*Fz)*(0.015*Fz + 67.7)*(kappa - 1.57e-6*Fz + 6.66e-4))/(2.71*Fz*LMU + 0.01)) - (0.7*Fz*exp(0.0135 - 1.35e-5*Fz)*(0.015*Fz + 67.7)*(kappa - 1.57e-6*Fz + 6.66e-4))/(2.71*Fz*LMU + 0.01)) - (0.7*Fz*exp(0.0135 - 1.35e-5*Fz)*(0.015*Fz + 67.7)*(kappa - 1.57e-6*Fz + 6.66e-4))/(2.71*Fz*LMU + 0.01))^2 + 1.0))
function u_ij = tc(u_max_old,vx,Fz,kappa)
fx = -(1.0*cos(0.989*atan((atan(0.159/(635.0*kappa^2 + 1.0)^(1/2)) - 0.159/(635.0*kappa^2 + 1.0)^(1/2))*(2.08e-4*Fz + 0.117) - 0.159/(635.0*kappa^2 + 1.0)^(1/2)))*(1.0e-4*Fz^2*LMU - 1.92*Fz*LMU*sin(1.41*atan((4.17e-5*Fz - 0.46)*(0.524*sign(kappa - 1.57e-6*Fz + 6.66e-4) + 1.0)*(atan((0.7*Fz*exp(0.0135 - 1.35e-5*Fz)*(0.015*Fz + 67.7)*(kappa - 1.57e-6*Fz + 6.66e-4))/(2.71*Fz*LMU + 0.01)) - (0.7*Fz*exp(0.0135 - 1.35e-5*Fz)*(0.015*Fz + 67.7)*(kappa - 1.57e-6*Fz + 6.66e-4))/(2.71*Fz*LMU + 0.01)) - (0.7*Fz*exp(0.0135 - 1.35e-5*Fz)*(0.015*Fz + 67.7)*(kappa - 1.57e-6*Fz + 6.66e-4))/(2.71*Fz*LMU + 0.01))))*(rs^2/Iw - 0.0148*kappa + 0.0148))/(vx*cos(0.989*atan((atan(0.159/(635.0*kappa^2 + 1.0)^(1/2)) - 0.159/(635.0*kappa^2 + 1.0)^(1/2))*(2.08e-4*Fz + 0.117) - 0.159/(635.0*kappa^2 + 1.0)^(1/2))));
delta_kappa = 0.001;
kappa_plus = kappa + delta_kappa;
fx_plus = -(1.0*cos(0.989*atan((atan(0.159/(635.0*kappa_plus^2 + 1.0)^(1/2)) - 0.159/(635.0*kappa_plus^2 + 1.0)^(1/2))*(2.08e-4*Fz + 0.117) - 0.159/(635.0*kappa_plus^2 + 1.0)^(1/2)))*(1.0e-4*Fz^2*LMU - 1.92*Fz*LMU*sin(1.41*atan((4.17e-5*Fz - 0.46)*(0.524*sign(kappa_plus - 1.57e-6*Fz + 6.66e-4) + 1.0)*(atan((0.7*Fz*exp(0.0135 - 1.35e-5*Fz)*(0.015*Fz + 67.7)*(kappa_plus - 1.57e-6*Fz + 6.66e-4))/(2.71*Fz*LMU + 0.01)) - (0.7*Fz*exp(0.0135 - 1.35e-5*Fz)*(0.015*Fz + 67.7)*(kappa_plus - 1.57e-6*Fz + 6.66e-4))/(2.71*Fz*LMU + 0.01)) - (0.7*Fz*exp(0.0135 - 1.35e-5*Fz)*(0.015*Fz + 67.7)*(kappa_plus - 1.57e-6*Fz + 6.66e-4))/(2.71*Fz*LMU + 0.01))))*(rs^2/Iw - 0.0148*kappa_plus + 0.0148))/(vx*cos(0.989*atan((atan(0.159/(635.0*kappa_plus^2 + 1.0)^(1/2)) - 0.159/(635.0*kappa_plus^2 + 1.0)^(1/2))*(2.08e-4*Fz + 0.117) - 0.159/(635.0*kappa_plus^2 + 1.0)^(1/2))));

Astar = (fx_plus - fx)/delta_kappa;

A = (1 + Astar*dt);

% ~~~~~~~~~~~~~~~~~~~~~~~~~~~~~~~~~~~~~~~~~~~~~~~~~~~~~~~~~~~~~~~~~~~~~~~ %
kappa_ref = 0.1;

% Q = 1e6;
Q = 5e5;
R = 0e-5;

u_ij = u_max_old + (B*Q*B + R)*( (Q*B)*kappa_ref - (A*Q*B)*kappa )/tau;
end

== matlab function TVModel_Simulation_21/Subsystem/Subsystem1/Slip Control/Traction Control/TC/Mu Linearization ==
  data: kappa input; mu0 output; mu1 output; Fz input; a0 output
function [mu0,mu1,a0] = fcn(kappa,Fz)

LMUX = 0.93;
J_wheel = 2e5/1e6;
rs = 0.235;
m = 270/4;
tau = 13.5;
dt = 0.02;

deltaKappa = 0.01;
kappa_plus = kappa + deltaKappa;

mu0 = muX(kappa,Fz,LMUX);
mu1 = (muX(kappa_plus,Fz,LMUX)-mu0)./(deltaKappa);

a0 = Fz./vx*mu1( (1-kappa)/m + rs^2/J_wheel );

end
function mu = muX(kappa,Fz,LMUX)
    mu = ((Fz.^2.*LMUX)./1.0e+4-Fz.*LMUX.*sin(atan((Fz.*5.946e-5-6.5736e-1).*(sign(Fz.*(-1.5696e-6)+kappa+6.665e-4).*5.242e-1+1.0).*(atan((Fz.*exp(Fz.*(-1.3455e-5)+1.3455e-2).*(Fz.*(3.0./2.0e+2)+6.77e+2./1.0e+1).*(Fz.*(-1.5696e-6)+kappa+6.665e-4).*(3.33e+2./4.0e+2))./(Fz.*LMUX.*2.5847808+1.0./1.0e+2))-(Fz.*exp(Fz.*(-1.3455e-5)+1.3455e-2).*(Fz.*(3.0./2.0e+2)+6.77e+2./1.0e+1).*(Fz.*(-1.5696e-6)+kappa+6.665e-4).*(3.33e+2./4.0e+2))./(Fz.*LMUX.*2.5847808+1.0./1.0e+2))-(Fz.*exp(Fz.*(-1.3455e-5)+1.3455e-2).*(Fz.*(3.0./2.0e+2)+6.77e+2./1.0e+1).*(Fz.*(-1.5696e-6)+kappa+6.665e-4).*(3.33e+2./4.0e+2))./(Fz.*LMUX.*2.5847808+1.0./1.0e+2)).*(1.68e+2./1.25e+2)).*1.9232)./Fz;
end

== stateflow chart TVModel_Simulation_21/Subsystem/Subsystem1/Slip Control/Traction Control/TC/Subsystem/Chart ==
  state OFF
    en,du:
    TC_max = [21];
  state ON
    en,du:
    TC_max = T_ff ;
  state SWITCHING_FILTER
    en,du:
    TC_max = TC_filter_tau*TC_max;
  (default) -> OFF
  OFF -> ON : [epsilon == 1]
  SWITCHING_FILTER -> ON [order 2] : [ epsilon == 1]
  SWITCHING_FILTER -> OFF [order 1] : [count(in(SWITCHING_FILTER)) > TC_filter_time/ts]
  ON -> SWITCHING_FILTER : [epsilon == 0]
  data: T_ff input; TC_max output; ts constant double =TV.MPC.T; TC_filter_time constant double =TV.MPC.mz_filter_time; TC_filter_tau constant double =TV.MPC.mz_filter_tau; epsilon input

== stateflow chart TVModel_Simulation_21/Subsystem/Subsystem1/Slip Control/Traction Control/TC/Subsystem/Chart1 ==
  state OFF
    en,du:
    TC_max = [21];
  state ON
    en,du:
    TC_max = T_ff ;
  state SWITCHING_FILTER
    en,du:
    TC_max = TC_filter_tau*TC_max;
  (default) -> OFF
  OFF -> ON : [epsilon == 1]
  SWITCHING_FILTER -> ON [order 2] : [ epsilon == 1]
  SWITCHING_FILTER -> OFF [order 1] : [count(in(SWITCHING_FILTER)) > TC_filter_time/ts]
  ON -> SWITCHING_FILTER : [epsilon == 0]
  data: T_ff input; TC_max output; ts constant double =TV.MPC.T; TC_filter_time constant double =TV.MPC.mz_filter_time; TC_filter_tau constant double =TV.MPC.mz_filter_tau; epsilon input

== stateflow chart TVModel_Simulation_21/Subsystem/Subsystem1/Slip Control/Traction Control/TC/Subsystem/Chart2 ==
  state OFF
    en,du:
    TC_max = [21];
  state ON
    en,du:
    TC_max = T_ff ;
  state SWITCHING_FILTER
    en,du:
    TC_max = TC_filter_tau*TC_max;
  (default) -> OFF
  OFF -> ON : [epsilon == 1]
  SWITCHING_FILTER -> ON [order 2] : [ epsilon == 1]
  SWITCHING_FILTER -> OFF [order 1] : [count(in(SWITCHING_FILTER)) > TC_filter_time/ts]
  ON -> SWITCHING_FILTER : [epsilon == 0]
  data: T_ff input; TC_max output; ts constant double =TV.MPC.T; TC_filter_time constant double =TV.MPC.mz_filter_time; TC_filter_tau constant double =TV.MPC.mz_filter_tau; epsilon input

== stateflow chart TVModel_Simulation_21/Subsystem/Subsystem1/Slip Control/Traction Control/TC/Subsystem/Chart3 ==
  state OFF
    en,du:
    TC_max = [21];
  state ON
    en,du:
    TC_max = T_ff ;
  state SWITCHING_FILTER
    en,du:
    TC_max = TC_filter_tau*TC_max;
  (default) -> OFF
  OFF -> ON : [epsilon == 1]
  SWITCHING_FILTER -> ON [order 2] : [ epsilon == 1]
  SWITCHING_FILTER -> OFF [order 1] : [count(in(SWITCHING_FILTER)) > TC_filter_time/ts]
  ON -> SWITCHING_FILTER : [epsilon == 0]
  data: T_ff input; TC_max output; ts constant double =TV.MPC.T; TC_filter_time constant double =TV.MPC.mz_filter_time; TC_filter_tau constant double =TV.MPC.mz_filter_tau; epsilon input

== matlab function TVModel_Simulation_21/Subsystem/Subsystem1/Slip Control/Traction Control/ABS/MATLAB Function1 ==
  data: vx input; T output; kappa input; Fz input; IN input; omega_p input; alpha input
function T = fcn(vx,kappa,Fz,IN,omega_p,alpha)

LMU = 0.8;
J_wheel = 2e5/1e6;
rs = 0.235;
m = 270/4;
tau = 13.5;
dt = 0.02;
g = 9.81;

% @(Fz,LMUX,kappa)
% Old tire
% muX = ((Fz.^2.*LMUX)./1.0e+4-Fz.*LMUX.*sin(atan((Fz.*5.946e-5-6.5736e-1).*(sign(Fz.*(-1.5696e-6)+kappa+6.665e-4).*5.242e-1+1.0).*(atan((Fz.*exp(Fz.*(-1.3455e-5)+1.3455e-2).*(Fz.*(3.0./2.0e+2)+6.77e+2./1.0e+1).*(Fz.*(-1.5696e-6)+kappa+6.665e-4).*(3.33e+2./4.0e+2))./(Fz.*LMUX.*2.5847808+1.0./1.0e+2))-(Fz.*exp(Fz.*(-1.3455e-5)+1.3455e-2).*(Fz.*(3.0./2.0e+2)+6.77e+2./1.0e+1).*(Fz.*(-1.5696e-6)+kappa+6.665e-4).*(3.33e+2./4.0e+2))./(Fz.*LMUX.*2.5847808+1.0./1.0e+2))-(Fz.*exp(Fz.*(-1.3455e-5)+1.3455e-2).*(Fz.*(3.0./2.0e+2)+6.77e+2./1.0e+1).*(Fz.*(-1.5696e-6)+kappa+6.665e-4).*(3.33e+2./4.0e+2))./(Fz.*LMUX.*2.5847808+1.0./1.0e+2)).*(1.68e+2./1.25e+2)).*1.9232)./Fz;

% New tire
% muX = (1.0e-4.*Fz.^2.*LMU - 1.92.*Fz.*LMU.*sin(1.41.*atan(0.7.*(5.95e-5.*Fz - 0.657).*(0.524*sign(kappa - 1.57e-6.*Fz + 6.66e-4) + 1.0).*(atan((0.7.*Fz.*exp(0.0135 - 1.35e-5.*Fz).*(0.015.*Fz + 67.7).*(kappa - 1.57e-6.*Fz + 6.66e-4))./(2.71.*Fz.*LMU + 0.01)) - (0.7.*Fz.*exp(0.0135 - 1.35e-5.*Fz).*(0.015.*Fz + 67.7).*(kappa - 1.57e-6.*Fz + 6.66e-4))./(2.71.*Fz.*LMU + 0.01)) - (0.7.*Fz.*exp(0.0135 - 1.35e-5.*Fz).*(0.015.*Fz + 67.7).*(kappa - 1.57e-6.*Fz + 6.66e-4))./(2.71.*Fz.*LMU + 0.01))))./Fz;
% alpha = zeros(4,1);

muX_com = abs((cos(0.989.*atan((23.4.*(alpha - 0.00681))./(635.0.*kappa.^2 + 1.0).^(1/2) - 1.0.*(atan((23.4.*(alpha - 0.00681))./(635.0.*kappa.^2 + 1.0).^(1/2)) - (23.4.*(alpha - 0.00681))./(635.0.*kappa.^2 + 1.0).^(1/2)).*(2.08e-4.*Fz + 0.117))).*(1.0e-4.*Fz.^2.*LMU - 1.92.*Fz.*LMU.*sin(1.41.*atan(0.7.*(5.95e-5.*Fz - 0.657).*(0.524.*sign(kappa - 1.57e-6.*Fz + 6.66e-4) + 1.0).*(atan((0.7.*Fz.*exp(0.0135 - 1.35e-5.*Fz).*(0.015.*Fz + 67.7).*(kappa - 1.57e-6.*Fz + 6.66e-4))./(2.71.*Fz.*LMU + 0.01)) - (0.7.*Fz.*exp(0.0135 - 1.35e-5.*Fz).*(0.015.*Fz + 67.7).*(kappa - 1.57e-6.*Fz + 6.66e-4))./(2.71.*Fz.*LMU + 0.01)) - (0.7.*Fz.*exp(0.0135 - 1.35e-5.*Fz).*(0.015.*Fz + 67.7).*(kappa - 1.57e-6.*Fz + 6.66e-4))./(2.71.*Fz.*LMU + 0.01)))))./(Fz.*cos(0.989.*atan((atan(0.159./(635.0.*kappa.^2 + 1.0).^(1/2)) - 0.159./(635.0.*kappa.^2 + 1.0).^(1/2)).*(2.08e-4.*Fz + 0.117) - 0.159./(635.0.*kappa.^2 + 1.0).^(1/2)))));

% T_fb = kappa_p/vx;
% kappa_lim = 0.1*ones(4,1);
% 
% for i = 1 : 4
%     if kappa(i) < kappa_lim(i)
%        T_fb(i) = 0;
%     end
% end

T= (IN + ( (1-kappa)/m + rs^2/J_wheel ).*Fz.*muX_com).*J_wheel/rs/tau;

% eta = - omega_p*rs/g;

% T_ff_deceleration = (+rs.^2./J_wheel./g.*muX.*Fz - eta).*J_wheel.*g/rs/tau/2;

% alpha = 0.96;
% alpha = 1;

% T_ff = T_ff_slip*alpha + T_ff_deceleration*(1 - alpha);

end

== matlab function TVModel_Simulation_21/Subsystem/Subsystem1/Slip Control/Traction Control/ABS/MATLAB Function2 ==
  data: T_max_controller input; T_max output; slip input; T_actual input; T_max_old input
function T_max = fcn(T_max_controller,slip,T_actual,T_max_old)

slip_target = -0.1*ones(4,1);
sDeact = 0.75;
T_max = zeros(4,1);

for i = 1:4 
    
    if slip(i) < slip_target(i)
        T_max(i) = T_max_controller(i);
    elseif T_actual(i) > T_max_old(i)*sDeact - 0.1;
        T_max(i) = T_max_old(i)-1;
        if T_max(i) < -21
           T_max(i) = -21;
        end
    else
        T_max(i) = T_max_controller(i);
    end
    
end

== matlab function TVModel_Simulation_21/Subsystem/Subsystem1/Slip Control/Traction Control/ABS/MATLAB Function3 ==
  data: T_old input; T_max output; omega_dot input; alpha input; T_brk input
function T_max = fcn(T_old,omega_dot,alpha,T_brk)

rs = 0.235;
M = 270/4;
Iw = 2e5/1e6;
tau = 13.5;

T_old = T_old.*tau;

Vw_dot = omega_dot.*rs;
Fd = -T_brk./rs + T_old./rs - Iw.*Vw_dot/(rs^2);

% alpha = 0.9;

T_max = (Iw./(alpha.*M*(rs).^2) + 1).*rs.*Fd;

T_max = T_max./tau;

for i = 1 : length(T_old)
    if T_old(i)/tau > -5
       T_max(i) = -21;
    end
end
